simulink model "Wheel_Control_Model"  (R2023b)
settings: Solver=FixedStepDiscrete  StartTime=0.0  StopTime=10.0  RelTol=1e-3
settings Model: Creator=E8KUAVE  LastModifiedBy=E8KUAVE
settings OptimizationCC: DefaultParameterBehavior=Inlined  EnhancedBackFolding=on  PassReuseOutputArgsAs=Individual arguments  ZeroExternalMemoryAtStartup=off  ZeroInternalMemoryAtStartup=off  OptimizeBlockOrder=speed  DifferentSizesBufferReuse=on  OptimizationCustomize=off  EfficientTunableParamExpr=on
settings DebuggingCC: ParameterTunabilityLossMsg=error
settings HardwareCC: ProdBitPerPointer=32  ProdBitPerSizeT=32  ProdBitPerPtrDiffT=32  ProdLargestAtomicInteger=Long  ProdLargestAtomicFloat=Double  ProdWordSize=32  ProdHWDeviceType=ARM Compatible->ARM Cortex-M
settings SFSimCC: MATLABDynamicMemAlloc=off  SimTargetLang=C++
settings RTWCC: Description=Embedded Coder  SystemTargetFile=ert.tlc  GenCodeOnly=on  TemplateMakefile=ert_default_tmf  Toolchain=MinGW64 | gmake (64-bit Windows)  DataTypeReplacement=CDataTypesFixedWidth  TargetLang=C++
settings CodeAppCC: ForceParamTrailComments=on  IgnoreCustomStorageClasses=off  OperatorAnnotations=on  SimulinkDataObjDesc=on  SFDataObjDesc=on  InsertBlockDesc=on
settings ERTTargetCC: TargetLangStandard=C++11 (ISO)  GenerateSampleERTMain=on  CodeInterfacePackaging=C++ class  PurelyIntegerCode=on  SupportNonFinite=off  InlinedParameterPlacement=NonHierarchical  RootIOFormat=Structure reference  ERTCustomFileTemplate=example_file_process.tlc  MaxIdInt64=INT64_MAX  MinIdInt64=INT64_MIN  MaxIdUint64=UINT64_MAX  MaxIdInt32=INT32_MAX  MinIdInt32=INT32_MIN  MaxIdUint32=UINT32_MAX  MaxIdInt16=INT16_MAX  MinIdInt16=INT16_MIN  MaxIdUint16=UINT16_MAX  MaxIdInt8=INT8_MAX  MinIdInt8=INT8_MIN  MaxIdUint8=UINT8_MAX

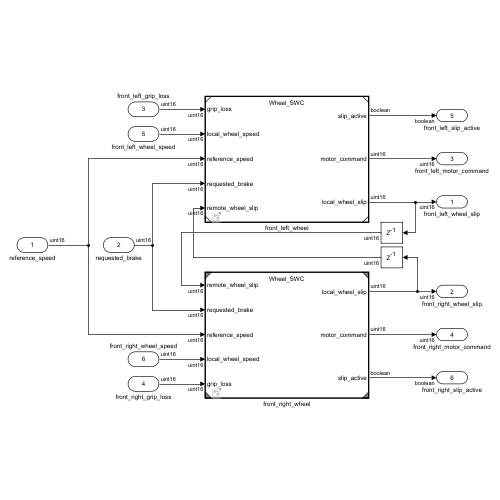
[thumbnail: Simulink's stored preview of the top-level diagram]
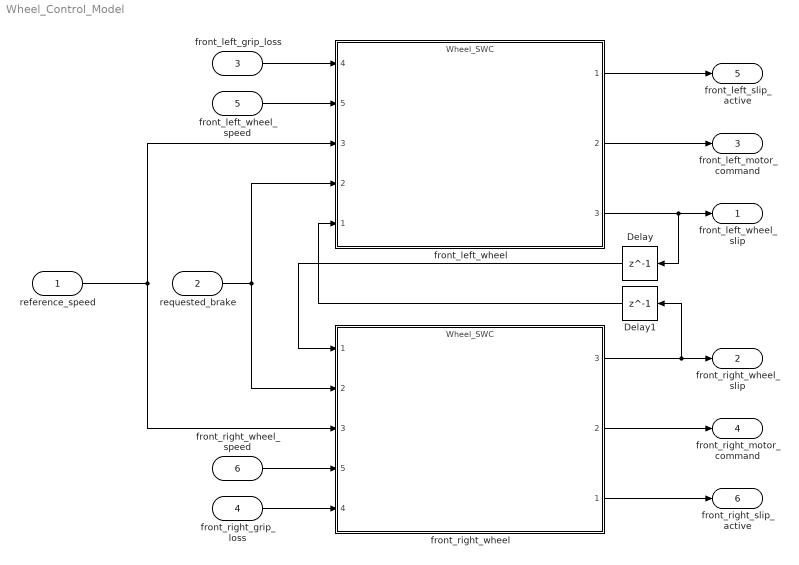
== system Wheel_Control_Model ==
  reference_speed : Inport  OutDataTypeStr=uint16
  requested_brake : Inport  Port=2  OutDataTypeStr=uint16
  front_left_grip_loss : Inport  Port=3  OutDataTypeStr=uint16
  front_right_grip_loss : Inport  Port=4  OutDataTypeStr=uint16
  front_left_wheel_speed : Inport  Port=5  OutDataTypeStr=uint16
  front_right_wheel_speed : Inport  Port=6  OutDataTypeStr=uint16
  Delay : Delay  DelayLength=1  InitialCondition=0
  Delay1 : Delay  DelayLength=1  InitialCondition=0
  front_left_wheel : ModelReference  ModelNameDialog=Wheel_SWC.slx  SimulationMode=Normal  ModelReferenceVersion=1.13
      settings: PortSchema="{\"entries\":[{\"content\":{\"sides\":[{\"content\":{\"connectorIds\":[\"In4\",\"In5\",\"In3\",\"In2\",\"In1\"]},\"type\":\"ConnectorPlacement.EquallySpacedRectSide\",\"uuid\":\"84a5f8d8-380d-4086-8686-6504858634fc\"},{\"content\":{\"connectorIds\":[\"Out1\",\"Out2\",\"Out3\"],\"side\":\"RIGHT\"},\"type\":\"ConnectorPlacement.EquallySpacedRectSide\",\"uuid\":\"3377f245-465b-4a90-a8d9-b33d2a559531\"},{\"content\":{\"side\":\"TOP\"},\"type\":\"ConnectorPlacement.EquallySpacedRectSide\",\"uuid\":\"850d46b7-1c57-4e1d-9f7a-30fff3f67c60\"}]},\"type\":\"ConnectorPlacement.EquallySpacedConnector\",\"uuid\":\"74bbaf4d-49e3-4915-8fa8-0bf568be98df\"}],\"packageUris\":[\"http://schema.mathworks.com/mf0/Connector/R2020b\"],\"version\":\"1.0\"}"
  front_right_wheel : ModelReference  ModelNameDialog=Wheel_SWC.slx  SimulationMode=Normal  ModelReferenceVersion=1.13
      settings: PortSchema="{\"entries\":[{\"content\":{\"sides\":[{\"content\":{\"connectorIds\":[\"In1\",\"In2\",\"In3\",\"In5\",\"In4\"]},\"type\":\"ConnectorPlacement.EquallySpacedRectSide\",\"uuid\":\"84a5f8d8-380d-4086-8686-6504858634fc\"},{\"content\":{\"connectorIds\":[\"Out3\",\"Out2\",\"Out1\"],\"side\":\"RIGHT\"},\"type\":\"ConnectorPlacement.EquallySpacedRectSide\",\"uuid\":\"3377f245-465b-4a90-a8d9-b33d2a559531\"},{\"content\":{\"side\":\"TOP\"},\"type\":\"ConnectorPlacement.EquallySpacedRectSide\",\"uuid\":\"850d46b7-1c57-4e1d-9f7a-30fff3f67c60\"}]},\"type\":\"ConnectorPlacement.EquallySpacedConnector\",\"uuid\":\"74bbaf4d-49e3-4915-8fa8-0bf568be98df\"}],\"packageUris\":[\"http://schema.mathworks.com/mf0/Connector/R2020b\"],\"version\":\"1.0\"}"
  front_left_wheel_slip : Outport  OutDataTypeStr=uint16
  front_right_wheel_slip : Outport  Port=2  OutDataTypeStr=uint16
  front_left_motor_command : Outport  Port=3  OutDataTypeStr=uint16
  front_right_motor_command : Outport  Port=4  OutDataTypeStr=uint16
  front_left_slip_active : Outport  Port=5  OutDataTypeStr=boolean
  front_right_slip_active : Outport  Port=6  OutDataTypeStr=boolean
  wires:
  reference_speed/1 -> front_right_wheel/3, front_left_wheel/3
  front_left_wheel_speed/1 -> front_left_wheel/5
  front_right_wheel_speed/1 -> front_right_wheel/5
  requested_brake/1 -> front_right_wheel/2, front_left_wheel/2
  front_left_grip_loss/1 -> front_left_wheel/4
  front_right_wheel/3 -> front_right_wheel_slip/1, Delay1/1
  front_left_wheel/3 -> front_left_wheel_slip/1, Delay/1
  front_right_grip_loss/1 -> front_right_wheel/4
  front_left_wheel/2 -> front_left_motor_command/1
  front_right_wheel/2 -> front_right_motor_command/1
  Delay1/1 -> front_left_wheel/1
  Delay/1 -> front_right_wheel/1
  front_left_wheel/1 -> front_left_slip_active/1
  front_right_wheel/1 -> front_right_slip_active/1
